simulink model "Y_DFK"  (R2013a)
settings: Solver=ode45  StartTime=0.0  StopTime=inf  RelTol=1e-3
undefined symbols (not defined in the file or in its folder): ToSimulink_Y_DFK_ST, ToSimulink_Y_Signals2VRML
libraries: vrlib x1
settings Model: Creator=Jose Angel Rangel  LastModifiedBy=Jose Angel Rangel

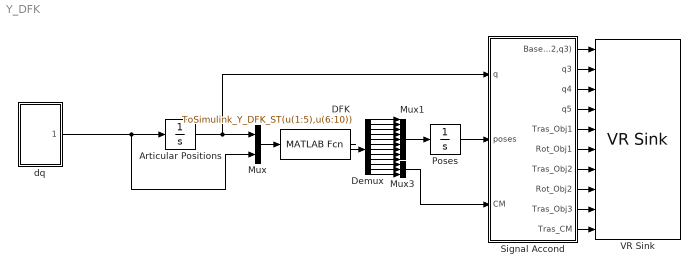
== system Y_DFK ==
  Articular Positions : Integrator
  DFK : MATLABFcn  MATLABFcn=ToSimulink_Y_DFK_ST(u(1:5),u(6:10))
  Demux : Demux  Outputs=12
  Mux : Mux  Inputs=2
  Mux1 : Mux  Inputs=9
  Mux3 : Mux  Inputs=3
  Poses : Integrator  InitialCondition=[-1.4142;3.4142;0;1.4142;3.4142;0;0;0;0]
  Signal Accond : Subsystem
  VR Sink : vrlib/VR Sink  InstantiateOnLoad=on  SampleTime=0.1  ViewEnable=on  RemoteChange=off  RemoteView=off  FieldsWritten=Base_Tras.translation.3.1.1.double#Base_Rot.rotation.4.1.1.double#Q4.rotation.4.1.1.double#Q5.rotation.4.1.1.double#Obj_RH.translation.3.1.1.double#Rot_Obj_RH.rotation.4.1.1.double#Obj_LH.translation.3.1.1.double#Rot_Obj_LH.rotation.4.1.1.double#Obj_CM.translation.3.1.1.double#Actual_CM.translation.3.1.1.double  WorldFileName=Simpley.wrl  AutoView=on  VideoDimensions=[]  AllowVariableSize=off
  dq : Subsystem
  wires:
  Mux/1 -> DFK/1
  DFK/1 -> Demux/1
  Demux/2 -> Mux1/2
  Demux/1 -> Mux1/1
  Demux/8 -> Mux1/8
  Demux/5 -> Mux1/5
  Demux/7 -> Mux1/7
  Demux/4 -> Mux1/4
  Demux/9 -> Mux1/9
  Demux/6 -> Mux1/6
  Demux/3 -> Mux1/3
  Demux/10 -> Mux3/1
  Demux/11 -> Mux3/2
  Demux/12 -> Mux3/3
  Mux1/1 -> Poses/1
  Articular Positions/1 -> Signal Accond/1(q), Mux/1
  Poses/1 -> Signal Accond/2(poses)
  Mux3/1 -> Signal Accond/3(CM)
  Signal Accond/2(q3) -> VR Sink/2
  Signal Accond/4(q5) -> VR Sink/4
  Signal Accond/3(q4) -> VR Sink/3
  Signal Accond/8(Rot_Obj2) -> VR Sink/8
  Signal Accond/6(Rot_Obj1) -> VR Sink/6
  Signal Accond/5(Tras_Obj1) -> VR Sink/5
  Signal Accond/7(Tras_Obj2) -> VR Sink/7
  Signal Accond/10(Tras_CM) -> VR Sink/10
  Signal Accond/9(Tras_Obj3) -> VR Sink/9
  Signal Accond/1(Base_Tras(q1,q2,q3)) -> VR Sink/1
  dq/1(Base config) -> Mux/2, Articular Positions/1

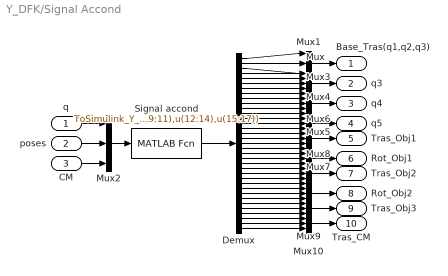
== system Y_DFK/Signal Accond ==
  q : Inport
  poses : Inport  Port=2
  CM : Inport  Port=3
  Demux : Demux  Outputs=35
  Mux{,3..5,7} (5 alike) : Mux
  Mux{1..2,6,8..10} (6 alike) : Mux  Inputs=3
  Signal accond : MATLABFcn  MATLABFcn=ToSimulink_Y_Signals2VRML(u(1:5),u(6:8),u(9:11),u(12:14),u(15:17))
  Base_Tras(q1,q2,q3) : Outport
  q3 : Outport  Port=2
  q4 : Outport  Port=3
  q5 : Outport  Port=4
  Tras_Obj1 : Outport  Port=5
  Rot_Obj1 : Outport  Port=6
  Tras_Obj2 : Outport  Port=7
  Rot_Obj2 : Outport  Port=8
  Tras_Obj3 : Outport  Port=9
  Tras_CM : Outport  Port=10
  wires:
  Mux2/1 -> Signal accond/1
  CM/1 -> Mux2/3
  poses/1 -> Mux2/2
  q/1 -> Mux2/1
  Signal accond/1 -> Demux/1
  Demux/13 -> Mux4/2
  Demux/5 -> Mux/2
  Demux/18 -> Mux6/3
  Demux/4 -> Mux/1
  Demux/3 -> Mux1/3
  Demux/9 -> Mux3/2
  Demux/10 -> Mux3/3
  Demux/14 -> Mux4/3
  Demux/12 -> Mux4/1
  Demux/7 -> Mux/4
  Demux/6 -> Mux/3
  Demux/8 -> Mux3/1
  Demux/11 -> Mux3/4
  Demux/17 -> Mux6/2
  Demux/16 -> Mux6/1
  Demux/15 -> Mux4/4
  Demux/1 -> Mux1/1
  Demux/2 -> Mux1/2
  Demux/21 -> Mux5/3
  Demux/22 -> Mux5/4
  Demux/24 -> Mux8/2
  Demux/23 -> Mux8/1
  Demux/19 -> Mux5/1
  Demux/20 -> Mux5/2
  Demux/25 -> Mux8/3
  Demux/28 -> Mux7/3
  Demux/29 -> Mux7/4
  Demux/26 -> Mux7/1
  Demux/35 -> Mux10/3
  Demux/30 -> Mux9/1
  Demux/34 -> Mux10/2
  Demux/33 -> Mux10/1
  Demux/27 -> Mux7/2
  Demux/31 -> Mux9/2
  Demux/32 -> Mux9/3
  Mux1/1 -> Base_Tras(q1,q2,q3)/1
  Mux/1 -> q3/1
  Mux3/1 -> q4/1
  Mux4/1 -> q5/1
  Mux6/1 -> Tras_Obj1/1
  Mux5/1 -> Rot_Obj1/1
  Mux8/1 -> Tras_Obj2/1
  Mux7/1 -> Rot_Obj2/1
  Mux9/1 -> Tras_Obj3/1
  Mux10/1 -> Tras_CM/1

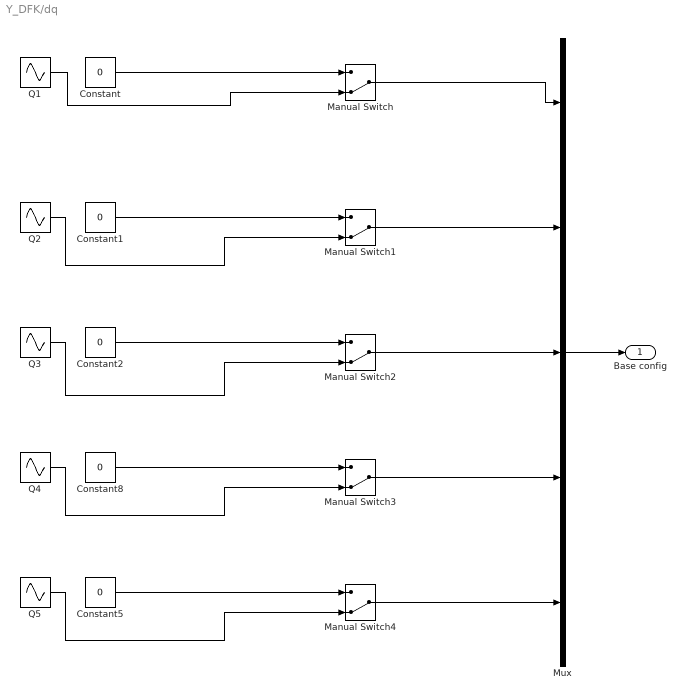
== system Y_DFK/dq ==
  Constant{,1..2,5,8} (5 alike) : Constant  Value=0
  Manual Switch{,1..4} (5 alike) : ManualSwitch  CurrentSetting=0
  Mux : Mux  Inputs=5
  Q1 : Sin  Amplitude=3.14  Frequency=.1  SampleTime=0
  Q2 : Sin  Amplitude=3.14  Frequency=.4  SampleTime=0
  Q3 : Sin  Amplitude=3.14  Frequency=.1  SampleTime=0
  Q4 : Sin  Amplitude=3.14  Frequency=.1  SampleTime=0
  Q5 : Sin  Amplitude=3.14  Frequency=.2  SampleTime=0
  Base config : Outport
  wires:
  Mux/1 -> Base config/1
  Manual Switch/1 -> Mux/1
  Q1/1 -> Manual Switch/2
  Constant/1 -> Manual Switch/1
  Manual Switch1/1 -> Mux/2
  Q2/1 -> Manual Switch1/2
  Constant1/1 -> Manual Switch1/1
  Manual Switch2/1 -> Mux/3
  Q3/1 -> Manual Switch2/2
  Constant2/1 -> Manual Switch2/1
  Manual Switch3/1 -> Mux/4
  Q4/1 -> Manual Switch3/2
  Constant8/1 -> Manual Switch3/1
  Manual Switch4/1 -> Mux/5
  Q5/1 -> Manual Switch4/2
  Constant5/1 -> Manual Switch4/1
